simulink model "Controlador_PID"  (R2025b)
settings: Solver=VariableStepAuto  StartTime=0.0  StopTime=10.0  RelTol=1e-3
undefined symbols (not defined in the file or in its folder): ctrller, scenario
libraries: slpidlib x1
settings Model: Creator=USUARIO  LastModifiedBy=USUARIO

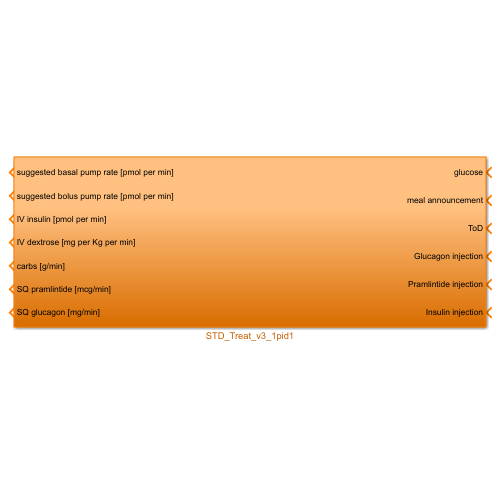
[thumbnail: Simulink's stored preview of the top-level diagram]
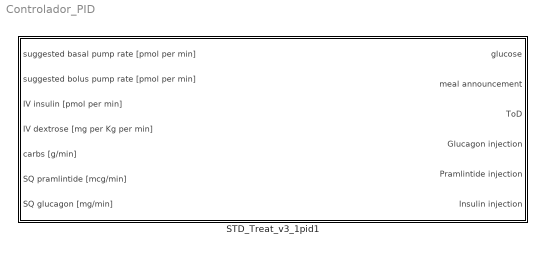
== system Controlador_PID ==
  STD_Treat_v3_1pid1 : Subsystem

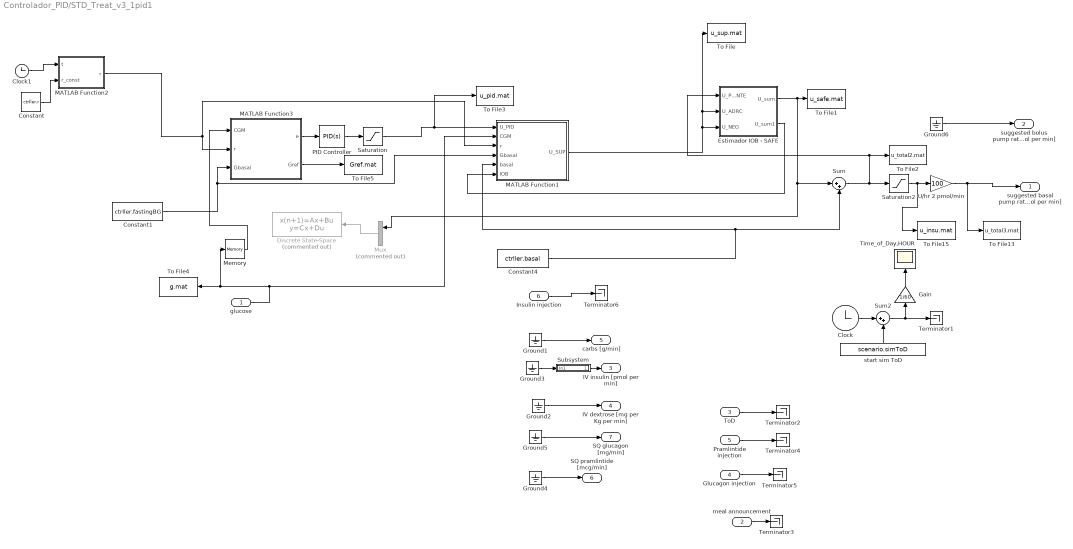
== system Controlador_PID/STD_Treat_v3_1pid1 ==
  glucose : Inport
  meal announcement : Inport  Port=2
  ToD : Inport  Port=3
  Glucagon injection : Inport  Port=4
  Pramlintide injection : Inport  Port=5
  Insulin injection : Inport  Port=6
  Clock : Clock
  Clock1 : Clock
  Constant : Constant  Value=ctrller.r
  Constant1 : Constant  Value=ctrller.fastingBG
  Constant4 : Constant  Value=ctrller.basal
  Discrete State-Space : DiscreteStateSpace  Commented=on  A=ctrller.KF.Aobs  B=ctrller.KF.Bobs  C=ctrller.KF.Cobs  D=ctrller.KF.Dobs  InitialCondition=ctrller.KF.x0  SampleTime=ctrller.KF.Ts
  Estimador IOB - SAFE : Subsystem
  Gain : Gain  Gain=1/60
  Ground{1..6} (6 alike) : Ground
  MATLAB Function1 : MATLAB Function  TreatAsAtomicUnit=on
  MATLAB Function2 : MATLAB Function  TreatAsAtomicUnit=on
  MATLAB Function3 : MATLAB Function  TreatAsAtomicUnit=on
  Memory : Memory
  Mux : Mux  Commented=on  Inputs=2
  PID Controller : slpidlib/PID Controller  Controller=PID  Form=Parallel  TimeDomain=Continuous-time  UseExternalTs=off  SampleTime=-1  IntegratorMethod=Forward Euler  FilterMethod=Forward Euler  ControllerParametersSource=internal  P=ctrller.p  I=ctrller.i  UseKiTs=off  D=ctrller.d  UseExternalDerivativeSource=off  N=100  UseFilter=on  TunerSelectOption=Transfer Function Based (PID Tuner App)  InitialConditionSource=internal  InitialConditionForIntegrator=0  InitialConditionForFilter=0  DifferentiatorICPrevScaledInput=0  ExternalReset=none  TrackingMode=off  Kt=1  LimitOutput=off  SatLimitsSource=internal  UpperSaturationLimit=inf  LowerSaturationLimit=-inf  LinearizeAsGain=on  AntiWindupMode=none  Kb=1  LimitIntegrator=off  UpperIntegratorSaturationLimit=inf  LowerIntegratorSaturationLimit=-inf  POutMin=[]  POutMax=[]  IOutMin=[]  IOutMax=[]  DOutMin=[]  DOutMax=[]  NOutMin=[]  NOutMax=[]  SumOutMin=[]  SumOutMax=[]  SaturationOutMin=[]  SaturationOutMax=[]  PParamMin=[]  PParamMax=[]  IParamMin=[]  IParamMax=[]  DParamMin=[]  DParamMax=[]  NParamMin=[]  NParamMax=[]  KbParamMin=[]  KbParamMax=[]  KtParamMin=[]  KtParamMax=[]  KbOutMin=[]  KbOutMax=[]  KtOutMin=[]  KtOutMax=[]  IntegratorOutMin=[]  IntegratorOutMax=[]  FilterOutMin=[]  FilterOutMax=[]  SumI1OutMin=[]  SumI1OutMax=[]  SumI2OutMin=[]  SumI2OutMax=[]  SumI3OutMin=[]  SumI3OutMax=[]  SumI4OutMin=[]  SumI4OutMax=[]  SumDOutMin=[]  SumDOutMax=[]  DifferentiatorOutMin=[]  DifferentiatorOutMax=[]  FilterDiffOutCoefMin=[]  FilterDiffOutCoefMax=[]  ReciprocalOutMin=[]  ReciprocalOutMax=[]  SumDenOutMin=[]  SumDenOutMax=[]  SumNumOutMin=[]  SumNumOutMax=[]  DivideOutMin=[]  DivideOutMax=[]  UdiffTsProdOutMin=[]  UdiffTsProdOutMax=[]  NTsProdOutMin=[]  NTsProdOutMax=[]  UintegralTsProdOutMin=[]  UintegralTsProdOutMax=[]  UngainTsProdOutMin=[]  UngainTsProdOutMax=[]  ClampingZeroOutDataTypeStr=Inherit: Inherit via back propagation  ClampingZeroOutMin=[]  ClampingZeroOutMax=[]  FilterDenConstantOutDataTypeStr=Inherit: Inherit via back propagation  FilterDenConstantOutMin=[]  FilterDenConstantOutMax=[]  PCopyOutDataTypeStr=Inherit: Inherit via back propagation  PCopyOutMin=[]  PCopyOutMax=[]  NCopyOutDataTypeStr=Inherit: Inherit via back propagation  NCopyOutMin=[]  NCopyOutMax=[]  IntegratorContinuousStateAttributes=''  IntegratorStateMustResolveToSignalObject=off  IntegratorRTWStateStorageClass=Auto  FilterContinuousStateAttributes=''  FilterStateMustResolveToSignalObject=off  FilterRTWStateStorageClass=Auto  ParallelPVariant=InternalParameters  IdealPVariant=Disabled  IVariant=InternalParameters  DVariant=InternalParameters  IntegratorVariant=Continuous  SatVariant=Disabled  AWVariant=Passthrough  PCopyVariant=Disabled  TRVariant=Disabled  FdbkBlocksVariant=Forward  IdealPFdbkVariant=Disabled  SatFdbkVariant=Disabled  DerivativeFilterVariant=ContFilter  NVariant=InternalParameters  NCopyVariant=Disabled  FilterICVariant=InternalICsFilter  IntegratorICVariant=InternalICs  ExternalResetVariant=Disabled  TRSumVariant=Passthrough  SumFdbkVariant=Disabled  SumVariant=Sum_PID  TsampFilterVariant=InternalTs  TsampNgainVariant=Passthrough  TsampIntegralVariant=Disabled_SignalSpec  ExternalSaturationOutDataTypeStr=Inherit: Same as second input  DerivativeSourceVariant=ErrorSignal  PreIntVariant=InternalPreInt
  Saturation : Saturate  UpperLimit=7  LowerLimit=-ctrller.basal
  Saturation2 : Saturate  UpperLimit=8  LowerLimit=0
  Subsystem : Subsystem
  Sum : Sum  Inputs=|++
  Sum2 : Sum  Inputs=|++
  Terminator{1..6} (6 alike) : Terminator
  Time_of_Day,HOUR : Scope
      settings: ActiveDisplayYMinimum=0  ActiveDisplayYMaximum=60000  DataLoggingVariableName=ScopeData22
  To File : ToFile  Filename=u_sup.mat  MatrixName=u_sup  SaveFormat=Timeseries
  To File1 : ToFile  Filename=u_safe.mat  MatrixName=u_safe  SaveFormat=Timeseries
  To File13 : ToFile  Filename=u_total3.mat  MatrixName=u_total3  SaveFormat=Timeseries
  To File15 : ToFile  Filename=u_insu.mat  MatrixName=u_insu  SaveFormat=Timeseries
  To File2 : ToFile  Filename=u_total2.mat  MatrixName=u_total2  SaveFormat=Timeseries
  To File3 : ToFile  Filename=u_pid.mat  MatrixName=u_pid  SaveFormat=Timeseries
  To File4 : ToFile  Filename=g.mat  MatrixName=g  SaveFormat=Timeseries
  To File5 : ToFile  Filename=Gref.mat  MatrixName=Gref  SaveFormat=Timeseries
  U/hr 2 pmol/min : Gain  Gain=100
  start sim ToD : Constant  Value=scenario.simToD
  suggested basal pump rate [pmol per min] : Outport
  suggested bolus pump rate [pmol per min] : Outport  Port=2
  IV insulin [pmol per min] : Outport  Port=3
  IV dextrose [mg per Kg per min] : Outport  Port=4
  carbs [g/min] : Outport  Port=5
  SQ pramlintide [mcg/min] : Outport  Port=6
  SQ glucagon [mg/min] : Outport  Port=7
  wires:
  Estimador IOB - SAFE/1(U_sum) -> To File1/1, Mux/1, Sum/1
  Sum/1 -> Saturation2/1, Estimador IOB - SAFE/1(U_PACIENTE), To File2/1
  Saturation/1 -> MATLAB Function1/1(U_PID), To File3/1
  MATLAB Function3/2(Gref) -> To File5/1
  MATLAB Function3/1(e) -> PID Controller/1
  glucose/1 -> MATLAB Function1/2(CGM), To File4/1, Memory/1
  Constant1/1 -> MATLAB Function1/4(Gbasal), MATLAB Function3/3(Gbasal)
  MATLAB Function2/1(r) -> MATLAB Function1/3(r), MATLAB Function3/2(r)
  PID Controller/1 -> Saturation/1
  Estimador IOB - SAFE/2(U_sum1) -> MATLAB Function1/6(IOB)
  meal announcement/1 -> Terminator3/1
  Saturation2/1 -> U/hr 2 pmol/min/1, To File15/1
  Constant/1 -> MATLAB Function2/2(r_const)
  Clock1/1 -> MATLAB Function2/1(t)
  MATLAB Function1/1(U_SUP) -> Estimador IOB - SAFE/3(U_NEG), Estimador IOB - SAFE/2(U_ADRC), To File/1
  Constant4/1 -> MATLAB Function1/5(basal), Sum/2
  Subsystem/1(IV insulin [pmol per min]) -> IV insulin [pmol per min]/1
  Ground3/1 -> Subsystem/1(In1)
  Insulin injection/1 -> Terminator6/1
  Ground1/1 -> carbs [g/min]/1
  Glucagon injection/1 -> Terminator5/1
  Ground2/1 -> IV dextrose [mg per Kg per min]/1
  Pramlintide injection/1 -> Terminator4/1
  Ground4/1 -> SQ pramlintide [mcg/min]/1
  Ground5/1 -> SQ glucagon [mg/min]/1
  Gain/1 -> Time_of_Day,HOUR/1
  start sim ToD/1 -> Sum2/2
  Sum2/1 -> Gain/1, Terminator1/1
  Clock/1 -> Sum2/1
  ToD/1 -> Terminator2/1
  U/hr 2 pmol/min/1 -> suggested basal pump rate [pmol per min]/1, To File13/1
  Ground6/1 -> suggested bolus pump rate [pmol per min]/1
  Mux/1 -> Discrete State-Space/1
  Memory/1 -> MATLAB Function3/1(CGM)

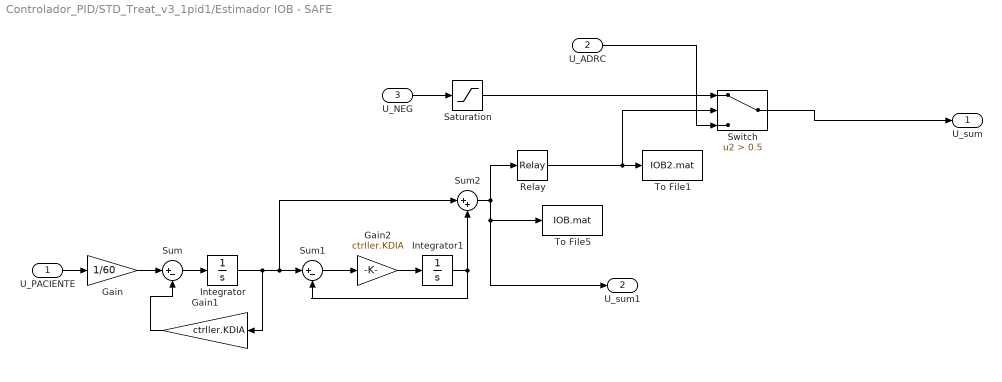
== system Controlador_PID/STD_Treat_v3_1pid1/Estimador IOB - SAFE ==
  U_PACIENTE : Inport
  U_ADRC : Inport  Port=2
  U_NEG : Inport  Port=3
  Gain : Gain  Gain=1/60
  Gain1 : Gain  Gain=ctrller.KDIA
  Gain2 : Gain  Gain=ctrller.KDIA
  Integrator : Integrator
  Integrator1 : Integrator
  Relay : Relay  OnSwitchValue=ctrller.sw  OffSwitchValue=ctrller.swneg
  Saturation : Saturate  UpperLimit=0  LowerLimit=-1000  ZeroCross=off
  Sum : Sum  Inputs=|+-
  Sum1 : Sum  Inputs=|+-
  Sum2 : Sum  Inputs=|++
  Switch : Switch  Criteria=u2 > Threshold  Threshold=0.5  SaturateOnIntegerOverflow=off  InputSameDT=off
  To File1 : ToFile  Filename=IOB2.mat  MatrixName=IOB2  SaveFormat=Timeseries
  To File5 : ToFile  Filename=IOB.mat  MatrixName=IOB  SaveFormat=Timeseries
  U_sum : Outport
  U_sum1 : Outport  Port=2
  wires:
  U_ADRC/1 -> Switch/3
  Saturation/1 -> Switch/1
  Switch/1 -> U_sum/1
  U_NEG/1 -> Saturation/1
  Relay/1 -> Switch/2, To File1/1
  Sum2/1 -> To File5/1, U_sum1/1, Relay/1
  Integrator1/1 -> Sum1/2, Sum2/2
  Gain2/1 -> Integrator1/1
  Sum1/1 -> Gain2/1
  Integrator/1 -> Gain1/1, Sum1/1, Sum2/1
  Gain1/1 -> Sum/2
  Sum/1 -> Integrator/1
  Gain/1 -> Sum/1
  U_PACIENTE/1 -> Gain/1

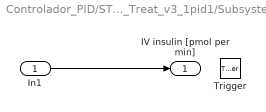
== system Controlador_PID/STD_Treat_v3_1pid1/Subsystem ==
  In1 : Inport
  Trigger : TriggerPort  VariantControl=(inherit)  PortDimensions=1
  IV insulin [pmol per min] : Outport
  wires:
  In1/1 -> IV insulin [pmol per min]/1

== matlab function Controlador_PID/STD_Treat_v3_1pid1/MATLAB Function1 ==
  data: U_PID input; U_SUP output; CGM input; r input; Gbasal input; basal input; IOB input
function U_SUP = Supervisor_PID(U_PID, CGM, r, Gbasal, basal, IOB)

%% =========================================================
% SUPERVISOR PARA CONTROLADOR PID + IOB
%
% Entradas:
%   U_PID  : accion correctiva generada por el PID [U/h]
%   CGM    : glucosa medida por el sensor [mg/dL]
%   r      : referencia como desviacion respecto a Gbasal
%            [mg/dL]
%   Gbasal : glucosa basal del paciente [mg/dL]
%   basal  : tasa basal de insulina del paciente [U/h]
%   IOB    : insulina activa estimada [U]
%
% Salida:
%   U_SUP  : accion correctiva supervisada [U/h]
%
% IMPORTANTE:
% U_SUP sigue siendo una CORRECCION respecto a la basal.
% La insulina basal se suma DESPUES de este bloque.
%
% Este supervisor no utiliza variables del ESO (z2, z3)
% ni variables persistentes.
%% =========================================================


%% =========================================================
% 1. RECONSTRUIR REFERENCIA ABSOLUTA
%% =========================================================

Gref = Gbasal + r;


%% =========================================================
% 2. PARAMETROS DEL SUPERVISOR
%% =========================================================

% Umbral absoluto de glucosa baja
G_low = 75.0;             % [mg/dL]

% Umbrales de IOB
IOB_soft = 3.5;           % [U]
IOB_med  = 4.5;           % [U]
IOB_high = 5.2;           % [U]


%% =========================================================
% 3. ERROR RESPECTO A LA REFERENCIA
%% =========================================================

error_glucosa = CGM - Gref;


%% =========================================================
% 4. SALIDA INICIAL
%% =========================================================

U_SUP = U_PID;


%% =========================================================
% 5. SEGURIDAD POR GLUCOSA BAJA
%
% Si CGM < 75 mg/dL, se solicita reducir casi
% completamente la basal.
%% =========================================================

if CGM < G_low

    U_SUP = -0.95 * basal;
    return

end


%% =========================================================
% 6. LIMITACION PROGRESIVA POR IOB
%
% Solo se limita una accion POSITIVA del PID.
% Las acciones negativas permanecen disponibles para
% reducir la administracion de insulina.
%% =========================================================

if U_SUP > 0

    if IOB >= IOB_high

        U_SUP = 0.20 * U_SUP;

    elseif IOB >= IOB_med

        U_SUP = 0.45 * U_SUP;

    elseif IOB >= IOB_soft

        U_SUP = 0.70 * U_SUP;

    end

end


%% =========================================================
% 7. PROTECCION ADICIONAL CERCA DE GLUCOSA BAJA
%
% Si la glucosa se encuentra por debajo de la referencia,
% no se permite una correccion positiva de insulina.
%
% Esto evita aumentar la administracion cuando la glucosa
% ya se encuentra por debajo del objetivo actual.
%% =========================================================

if error_glucosa < 0.0 && U_SUP > 0.0

    U_SUP = 0.0;

end

end

== matlab function Controlador_PID/STD_Treat_v3_1pid1/MATLAB Function2 ==
  data: t input; r output; r_const input
function r = referencia_horaria(t, r_const)

% t en minutos
% r_const viene de un bloque Constant

if t < 240
    r = 0;          % al inicio apunta a 122 mg/dL

elseif t < 360
    r = r_const*(t-240)/(360-240);  % transición suave

else
    r = r_const;    % referencia final
end

end

== matlab function Controlador_PID/STD_Treat_v3_1pid1/MATLAB Function3 ==
  data: e output; CGM input; r input; Gbasal input; Gref output
function [e, Gref] = Error_PID(CGM, r, Gbasal)

Gref = Gbasal + r;
e = CGM - Gref;

end
